simulink model "Active_Suspension_Control_Simulink_Fuzzy"  (R2023b)
settings: Solver=VariableStepAuto  StartTime=0.0  StopTime=10  MaxStep=1e-3  RelTol=1e-3
values from neighbouring files (symbols this model uses):
  a = [1 20 3486.66666667 10555.5555556 168888.888889]    [Fuzzy_Workspace.mat]    (also in quarter_car_model.m = 0.8)
  b = [0 0 0.00333333333333 10555.6111112 168900.333335]    [Fuzzy_Workspace.mat]
  c_car = 1000    [Active_Suspension_Control.m]    (also in Fuzzy_Workspace.mat)
  k_car = 16000    [Active_Suspension_Control.m]    (also in Fuzzy_Workspace.mat)
  k_wheel = 190000    [Active_Suspension_Control.m]    (also in Fuzzy_Workspace.mat)
  m_car = 300    [Active_Suspension_Control.m]    (also in Fuzzy_Workspace.mat)
  m_wheel = 60    [Active_Suspension_Control.m]    (also in Fuzzy_Workspace.mat)
libraries: fuzblock x1
settings Model: Creator=hkurt  LastModifiedBy=hkurt
settings SolverCC: ZeroCrossControl=DisableAll  EnableFixedStepZeroCrossing=on

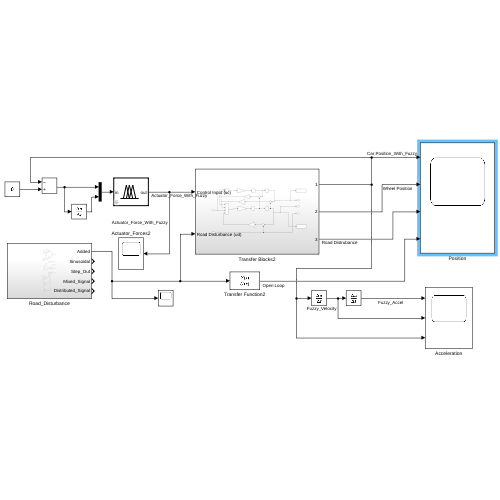
[thumbnail: Simulink's stored preview of the top-level diagram]
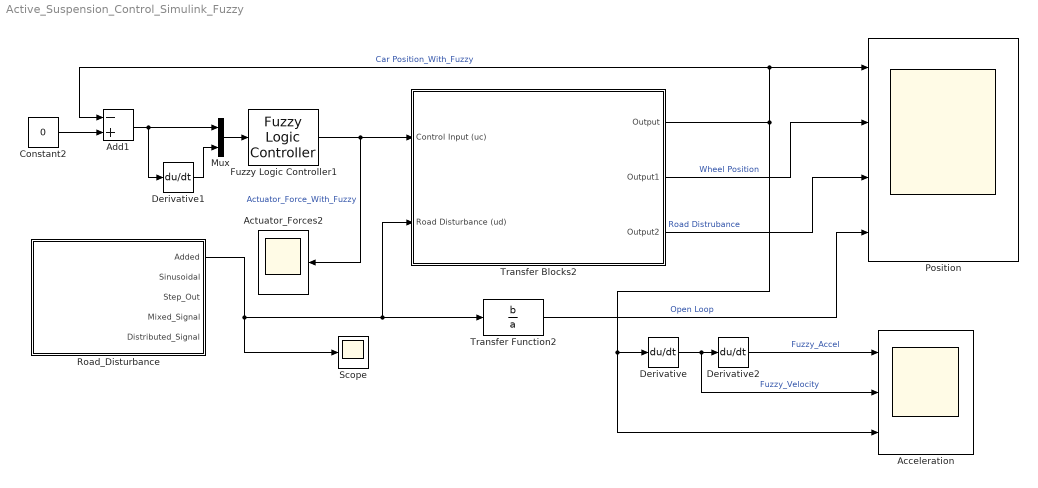
== system Active_Suspension_Control_Simulink_Fuzzy ==
  Acceleration : Scope  NumInputPorts=3
  Actuator_Forces2 : Scope
  Add1 : Sum  Inputs=-+
  Constant2 : Constant  Value=0
  Derivative : Derivative
  Derivative1 : Derivative
  Derivative2 : Derivative
  Fuzzy Logic Controller1 : fuzblock/Fuzzy Logic  Controller  FIS=my_fuzzy_4  OutputSampleNumber=101  DataType=double  FuzzifiedInputs=off  RuleFiringStrengths=off  RuleOutputs=off  AggregatedOutputs=off  SimulateUsing=Interpreted execution  OutOfRangeInputValueMessage=warning  NoRuleFiredMessage=warning  EmptyOutputFuzzySetMessage=warning
  Mux : Mux  Inputs=2
  Position : Scope  NumInputPorts=4
  Road_Disturbance : Subsystem
  Scope : Scope
  Transfer Blocks2 : Subsystem
  Transfer Function2 : TransferFcn  Numerator=b  Denominator=a
  wires:
  Transfer Function2/1 -> Position/4  "Open Loop"
  Transfer Blocks2/3(Output2) -> Position/3  "Road Distrubance"
  Transfer Blocks2/2(Output1) -> Position/2  "Wheel Position"
  Transfer Blocks2/1(Output) -> Acceleration/3, Derivative/1, Position/1, Add1/1  "Car Position_With_Fuzzy"
  Add1/1 -> Derivative1/1, Mux/1
  Mux/1 -> Fuzzy Logic Controller1/1
  Derivative1/1 -> Mux/2
  Constant2/1 -> Add1/2
  Fuzzy Logic Controller1/1 -> Transfer Blocks2/1(Control Input (uc)), Actuator_Forces2/1  "Actuator_Force_With_Fuzzy"
  Derivative/1 -> Acceleration/2, Derivative2/1  "Fuzzy_Velocity"
  Derivative2/1 -> Acceleration/1  "Fuzzy_Accel"
  Road_Disturbance/1(Added) -> Scope/1, Transfer Function2/1, Transfer Blocks2/2(Road Disturbance (ud))

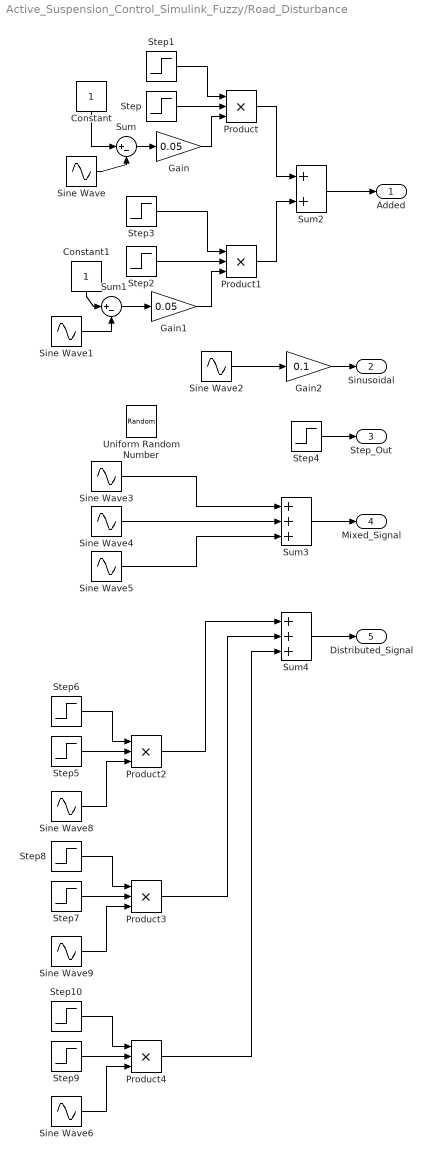
== system Active_Suspension_Control_Simulink_Fuzzy/Road_Disturbance ==
  Constant : Constant
  Constant1 : Constant
  Gain : Gain  Gain=0.05
  Gain1 : Gain  Gain=0.05
  Gain2 : Gain  Gain=0.1
  Product{,1..4} (5 alike) : Product  Inputs=3
  Sine Wave : Sin  Frequency=2*pi  Phase=pi*3/2  SampleTime=0
  Sine Wave1 : Sin  Frequency=2*pi  Phase=pi*3/2  SampleTime=0
  Sine Wave2 : Sin  Frequency=2*pi  Phase=pi  SampleTime=0
  Sine Wave3 : Sin  Amplitude=0.01  Frequency=15*pi  SampleTime=0
  Sine Wave4 : Sin  Amplitude=0.02  Frequency=10*pi  Phase=pi/2  SampleTime=0
  Sine Wave5 : Sin  Amplitude=0.03  Frequency=pi  SampleTime=0
  Sine Wave6 : Sin  Amplitude=0.08  Frequency=pi  Phase=pi*3/2  SampleTime=0
  Sine Wave8 : Sin  Amplitude=0.1  Frequency=pi  Phase=pi*3/2  SampleTime=0
  Sine Wave9 : Sin  Amplitude=0.05  Frequency=pi  Phase=pi*3/2  SampleTime=0
  Step : Step  Time=1.5  Before=1  After=0  SampleTime=0
  Step1 : Step  Time=0.5  SampleTime=0
  Step10 : Step  Time=8.5  SampleTime=0
  Step2 : Step  Time=3.5  Before=1  After=0  SampleTime=0
  Step3 : Step  Time=2.5  SampleTime=0
  Step4 : Step  Time=2  After=0.015  SampleTime=0
  Step5 : Step  Time=1.5  Before=1  After=0  SampleTime=0
  Step6 : Step  Time=0.5  SampleTime=0
  Step7 : Step  Time=5.5  Before=1  After=0  SampleTime=0
  Step8 : Step  Time=4.5  SampleTime=0
  Step9 : Step  Time=9.5  Before=1  After=0  SampleTime=0
  Sum : Sum  Inputs=|+-
  Sum1 : Sum  Inputs=|+-
  Sum2 : Sum
  Sum3 : Sum  Inputs=+++
  Sum4 : Sum  Inputs=+++
  Uniform Random Number : UniformRandomNumber  Minimum=-0.05  Maximum=0.05  SampleTime=0.1
  Added : Outport
  Sinusoidal : Outport  Port=2
  Step_Out : Outport  Port=3
  Mixed_Signal : Outport  Port=4
  Distributed_Signal : Outport  Port=5
  wires:
  Constant/1 -> Sum/1
  Step/1 -> Product/2
  Sum/1 -> Gain/1
  Gain/1 -> Product/3
  Sine Wave/1 -> Sum/2
  Step1/1 -> Product/1
  Gain1/1 -> Product1/3
  Step2/1 -> Product1/2
  Step3/1 -> Product1/1
  Product1/1 -> Sum2/2
  Product/1 -> Sum2/1
  Constant1/1 -> Sum1/1
  Sine Wave1/1 -> Sum1/2
  Sum1/1 -> Gain1/1
  Sine Wave2/1 -> Gain2/1
  Sum2/1 -> Added/1
  Gain2/1 -> Sinusoidal/1
  Step4/1 -> Step_Out/1
  Sum3/1 -> Mixed_Signal/1
  Sine Wave3/1 -> Sum3/1
  Sine Wave4/1 -> Sum3/2
  Sine Wave5/1 -> Sum3/3
  Step6/1 -> Product2/1
  Product2/1 -> Sum4/1
  Step5/1 -> Product2/2
  Sine Wave8/1 -> Product2/3
  Sum4/1 -> Distributed_Signal/1
  Step8/1 -> Product3/1
  Step7/1 -> Product3/2
  Sine Wave9/1 -> Product3/3
  Product3/1 -> Sum4/2
  Step10/1 -> Product4/1
  Step9/1 -> Product4/2
  Sine Wave6/1 -> Product4/3
  Product4/1 -> Sum4/3

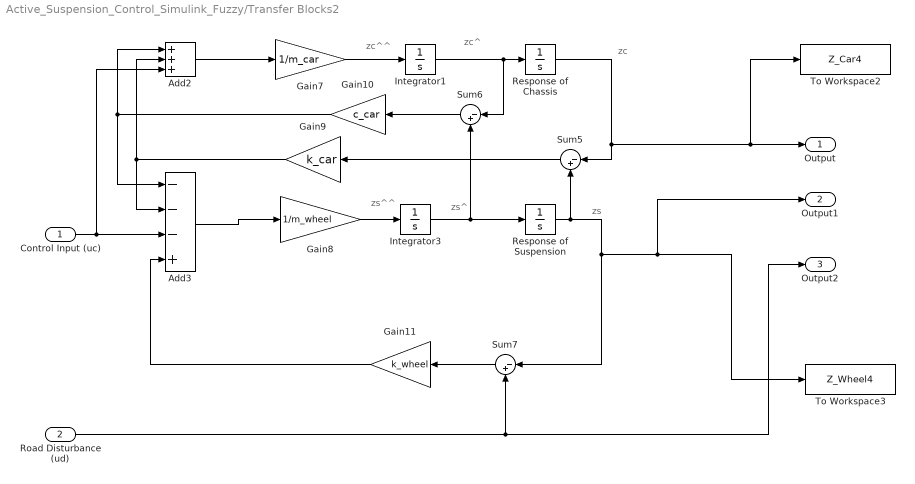
== system Active_Suspension_Control_Simulink_Fuzzy/Transfer Blocks2 ==
  note: zs
  note: zc^^
  note: zc
  note: zc^
  note: zs^^
  note: zs^
  Control Input (uc) : Inport
  Road Disturbance (ud) : Inport  Port=2
  Add2 : Sum  Inputs=+++
  Add3 : Sum  Inputs=---+
  Gain10 : Gain  Gain=c_car
  Gain11 : Gain  Gain=k_wheel
  Gain7 : Gain  Gain=1/m_car
  Gain8 : Gain  Gain=1/m_wheel
  Gain9 : Gain  Gain=k_car
  Integrator1 : Integrator
  Integrator3 : Integrator
  Response of Chassis : Integrator
  Response of Suspension : Integrator
  Sum5 : Sum  Inputs=|-+
  Sum6 : Sum  Inputs=|-+
  Sum7 : Sum  Inputs=|-+
  To Workspace2 : ToWorkspace  VariableName=Z_Car4  SaveFormat=Timeseries  SampleTime=-1
  To Workspace3 : ToWorkspace  VariableName=Z_Wheel4  SaveFormat=Timeseries  SampleTime=-1
  Output : Outport
  Output1 : Outport  Port=2
  Output2 : Outport  Port=3
  wires:
  Gain11/1 -> Add3/4
  Sum5/1 -> Gain9/1
  Add3/1 -> Gain8/1
  Response of Suspension/1 -> Sum5/2, Sum7/1, Output1/1, To Workspace3/1
  Sum7/1 -> Gain11/1
  Integrator1/1 -> Sum6/1, Response of Chassis/1
  Gain8/1 -> Integrator3/1
  Gain9/1 -> Add3/2, Add2/2
  Sum6/1 -> Gain10/1
  Response of Chassis/1 -> Sum5/1, Output/1, To Workspace2/1
  Gain7/1 -> Integrator1/1
  Road Disturbance (ud)/1 -> Sum7/2, Output2/1
  Integrator3/1 -> Sum6/2, Response of Suspension/1
  Add2/1 -> Gain7/1
  Gain10/1 -> Add3/1, Add2/1
  Control Input (uc)/1 -> Add2/3, Add3/3
